simulink model "Example_9_Code_Generation_Mdl"  (Simulink 7.8)
settings: Solver=ode45  StartTime=0.0  StopTime=15  RelTol=1e-3
values from neighbouring files (symbols this model uses):
  A = sys.a    [Example_2_Control.m]    (also in Example_2_Discretization.m; Example_2_Disturbance_Estimation.m; Example_2_Integral_Control.m; Example_2_Prediction_Observer.m)
  B = sys.b    [Example_2_Control.m]    (also in Example_2_Discretization.m; Example_2_Disturbance_Estimation.m; Example_2_Integral_Control.m; Example_2_Prediction_Observer.m)
  C = sys.c    [Example_2_Control.m]    (also in Example_2_Discretization.m; Example_2_Disturbance_Estimation.m; Example_2_Integral_Control.m; Example_2_Prediction_Observer.m)
  Ts = 1    [Example_9_Code_Generation.m]    (also in Example_9_Modeling_Simulation.m; Example_9_Regulation.m; Example_9_Tracking.m; Example_9_Tracking_Delta_Input_Formulation.m)
  x_0 = [0; 0; 0; 0]    [Example_2_Analysis.m]    (also in Example_2_Control.m = [25*9.81/k_s; 0; 25*9.81/k_u; 0]; Example_2_Discretization.m = [25*9.81/k_s; 0; 25*9.81/k_u; 0]; Example_2_Disturbance_Estimation.m; Example_2_Integral_Control.m)
undefined symbols (not defined in the file or in its folder): mycontroller_reduced
settings Model: Creator=d_goerges  LastModifiedBy=d_goerges
settings DataIOCC: SignalLoggingSaveFormat=Dataset
settings OptimizationCC: ExpressionDepthLimit=128
settings DebuggingCC: UnderspecifiedInitializationDetection=Simplified  MergeDetectMultiDrivingBlocksExec=error  SolverPrmCheckMsg=none  FrameProcessingCompatibilityMsg=error  StateNameClashWarn=none
settings CodeAppCC: CustomSymbolStrType=$N$R$M_T
settings GRTTargetCC: TargetFunctionLibrary=C89/C90 (ANSI)

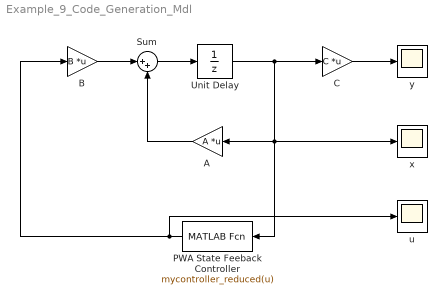
== system Example_9_Code_Generation_Mdl ==
  A : Gain  Gain=A  Multiplication=Matrix(K*u)
  B : Gain  Gain=B  Multiplication=Matrix(K*u)
  C : Gain  Gain=C  Multiplication=Matrix(K*u)
  PWA State Feeback Controller : MATLABFcn  MATLABFcn=mycontroller_reduced(u)
  Sum : Sum  Inputs=|++
  Unit Delay : UnitDelay  X0=x_0  SampleTime=Ts
  u : Scope
      settings: SaveName=ScopeData2
  x : Scope
  y : Scope
  wires:
  Unit Delay/1 -> C/1, x/1, PWA State Feeback Controller/1, A/1
  Sum/1 -> Unit Delay/1
  A/1 -> Sum/2
  B/1 -> Sum/1
  PWA State Feeback Controller/1 -> B/1, u/1
  C/1 -> y/1
